simulink model "PIDkh4_controller"  (R2020a)
settings: Solver=VariableStepAuto  StartTime=0.0  StopTime=40  RelTol=1e-3
libraries: simulink x2, dspinverses x1
settings Model: Creator=FlightControlLab  LastModifiedBy=javier
settings SolverCC: SolverResetMethod=Robust
settings DataIOCC: ReturnWorkspaceOutputs=off
settings DebuggingCC: ArithmeticOperatorsInVariantConditions=warning
settings SFSimCC: SimUseLocalCustomCode=off  CustomCodeUndefinedFunction=UseInterfaceOnly
settings RTWCC: RTWUseLocalCustomCode=off

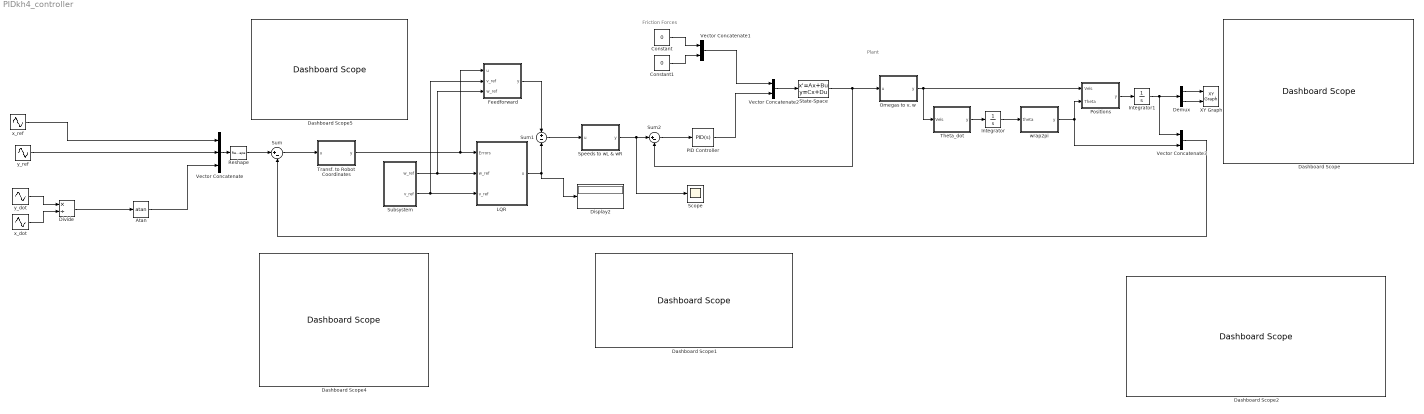
== system PIDkh4_controller ==
  note: Plant
  note: Friction Forces
  Atan : Trigonometry  Operator=atan
  Constant : Constant  Value=0
  Constant1 : Constant  Value=0
  Dashboard Scope{,1..2,4..5} (5 alike) : DashboardScope
  Demux : Demux  Outputs=2
  Display2 : Display
  Divide : Product  Inputs=*/
  Feedforward : MATLAB Function  TreatAsAtomicUnit=on
  Integrator : Integrator
  Integrator1 : Integrator
  LQR : Subsystem
  "Omegas to v, w" : MATLAB Function  TreatAsAtomicUnit=on
  PID Controller : simulink/Continuous/PID Controller  Controller=PID  Form=Parallel  TimeDomain=Continuous-time  UseExternalTs=off  SampleTime=-1  IntegratorMethod=Forward Euler  FilterMethod=Forward Euler  ControllerParametersSource=internal  P=10  I=10  D=1  UseFilter=on  N=100  TunerSelectOption=Transfer Function Based (PID Tuner App)  InitialConditionSource=internal  InitialConditionForIntegrator=0  InitialConditionForFilter=0  DifferentiatorICPrevScaledInput=0  ExternalReset=none  TrackingMode=off  Kt=1  LimitOutput=off  UpperSaturationLimit=inf  LowerSaturationLimit=-inf  LinearizeAsGain=on  AntiWindupMode=none  Kb=1  POutMin=[]  POutMax=[]  IOutMin=[]  IOutMax=[]  DOutMin=[]  DOutMax=[]  NOutMin=[]  NOutMax=[]  SumOutMin=[]  SumOutMax=[]  SaturationOutMin=[]  SaturationOutMax=[]  PParamMin=[]  PParamMax=[]  IParamMin=[]  IParamMax=[]  DParamMin=[]  DParamMax=[]  NParamMin=[]  NParamMax=[]  KbParamMin=[]  KbParamMax=[]  KtParamMin=[]  KtParamMax=[]  KbOutMin=[]  KbOutMax=[]  KtOutMin=[]  KtOutMax=[]  IntegratorOutMin=[]  IntegratorOutMax=[]  FilterOutMin=[]  FilterOutMax=[]  SumI1OutMin=[]  SumI1OutMax=[]  SumI2OutMin=[]  SumI2OutMax=[]  SumI3OutMin=[]  SumI3OutMax=[]  SumI4OutMin=[]  SumI4OutMax=[]  SumDOutMin=[]  SumDOutMax=[]  DifferentiatorOutMin=[]  DifferentiatorOutMax=[]  FilterDiffOutCoefMin=[]  FilterDiffOutCoefMax=[]  ReciprocalOutMin=[]  ReciprocalOutMax=[]  SumDenOutMin=[]  SumDenOutMax=[]  SumNumOutMin=[]  SumNumOutMax=[]  DivideOutMin=[]  DivideOutMax=[]  UdiffTsProdOutMin=[]  UdiffTsProdOutMax=[]  NTsProdOutMin=[]  NTsProdOutMax=[]  UintegralTsProdOutMin=[]  UintegralTsProdOutMax=[]  UngainTsProdOutMin=[]  UngainTsProdOutMax=[]  IntegratorContinuousStateAttributes=''  IntegratorStateMustResolveToSignalObject=off  IntegratorRTWStateStorageClass=Auto  FilterContinuousStateAttributes=''  FilterStateMustResolveToSignalObject=off  FilterRTWStateStorageClass=Auto  ParallelPVariant=InternalParameters  IdealPVariant=Disabled  IVariant=InternalParameters  DVariant=InternalParameters  IntegratorVariant=Continuous  SatVariant=Disabled  AWVariant=Passthrough  PCopyVariant=Disabled  TRVariant=Disabled  FdbkBlocksVariant=Forward  IdealPFdbkVariant=Disabled  SatFdbkVariant=Disabled  DerivativeFilterVariant=ContFilter  NVariant=InternalParameters  NCopyVariant=Disabled  FilterICVariant=InternalICsFilter  IntegratorICVariant=InternalICs  ExternalResetVariant=Disabled  TRSumVariant=Passthrough  SumFdbkVariant=Disabled  SumVariant=Sum_PID  TsampFilterVariant=InternalTs  TsampNgainVariant=Passthrough  TsampIntegralVariant=Passthrough
  Positions : MATLAB Function  TreatAsAtomicUnit=on
  Reshape : Reshape  OutputDimensionality=Column vector (2-D)
  Scope : Scope
  Speeds to wL & wR : MATLAB Function  TreatAsAtomicUnit=on
  State-Space : StateSpace  A=[0, 0, 0, 0; 0, 0, 0, 0; 0, 0, -0.0100, 0; 0, 0, 0, -0.0100]  B=[1.7699, 1.7699, 0, 0; 0.725, -0.725, 0, 0; -0.2100, 0, 10, 0; 0, -0.2100, 0, 10.0000]  C=[0, 0, 1, 0; 0, 0, 0, 1]  D=[0, 0, 0, 0; 0, 0, 0, 0]  InitialCondition=0
  Subsystem : Subsystem
  Sum : Sum  Inputs=|+-
  Sum1 : Sum  Inputs=+-
  Sum2 : Sum  Inputs=|+-
  Theta_dot : MATLAB Function  TreatAsAtomicUnit=on
  Transf. to Robot Coordinates : MATLAB Function  TreatAsAtomicUnit=on
  Vector Concatenate : Concatenate  NumInputs=3
  Vector Concatenate1 : Concatenate
  Vector Concatenate2 : Concatenate
  Vector Concatenate3 : Concatenate
  XY Graph : simulink/Sinks/XY Graph  xmin=-1  xmax=1  ymin=-1  ymax=1  st=-1
  wrap2pi : MATLAB Function  TreatAsAtomicUnit=on
  x_dot : Sin  Amplitude=0.3^2  Frequency=0.3  Phase=pi/2  SampleTime=0
  x_ref : Sin  Amplitude=0.3  Frequency=0.3  SampleTime=0
  y_dot : Sin  Amplitude=-0.3^2  Frequency=0.3  SampleTime=0
  y_ref : Sin  Amplitude=0.3  Bias=-0.3  Frequency=0.3  Phase=pi/2  SampleTime=0
  wires:
  x_ref/1 -> Vector Concatenate/1
  y_ref/1 -> Vector Concatenate/2
  Transf. to Robot Coordinates/1(y) -> LQR/1(Errors), Feedforward/1(u)
  Subsystem/1(w_ref) -> LQR/2(w_ref), Feedforward/3(w_ref)
  Sum1/1 -> Speeds to wL & wR/1(u)
  State-Space/1 -> Sum2/2, "Omegas to v, w"/1(u)
  Constant/1 -> Vector Concatenate1/1
  Constant1/1 -> Vector Concatenate1/2
  Vector Concatenate2/1 -> State-Space/1
  Vector Concatenate1/1 -> Vector Concatenate2/1
  Positions/1(y) -> Integrator1/1
  "Omegas to v, w"/1(y) -> Positions/1(Vels), Theta_dot/1(Vels)
  Theta_dot/1(y) -> Integrator/1
  Integrator1/1 -> Vector Concatenate3/1, Demux/1
  Vector Concatenate3/1 -> Sum/2
  Subsystem/2(v_ref) -> LQR/3(v_ref), Feedforward/2(v_ref)
  Vector Concatenate/1 -> Reshape/1
  Reshape/1 -> Sum/1
  Sum/1 -> Transf. to Robot Coordinates/1(u)
  Feedforward/1(y) -> Sum1/1
  y_dot/1 -> Divide/1
  x_dot/1 -> Divide/2
  Speeds to wL & wR/1(y) -> Scope/1, Sum2/1
  Sum2/1 -> PID Controller/1
  PID Controller/1 -> Vector Concatenate2/2
  LQR/1(u) -> Display2/1, Sum1/2
  Demux/1 -> XY Graph/1
  Demux/2 -> XY Graph/2
  Integrator/1 -> wrap2pi/1(theta)
  wrap2pi/1(y) -> Positions/2(Theta), Vector Concatenate3/2
  Atan/1 -> Vector Concatenate/3
  Divide/1 -> Atan/1

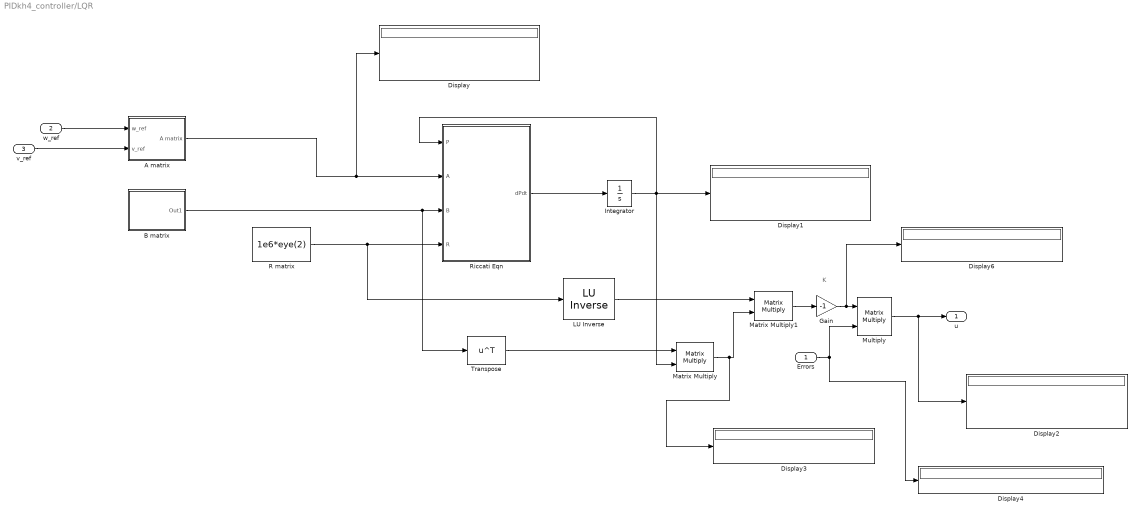
== system PIDkh4_controller/LQR ==
  note: K
  Errors : Inport
  w_ref : Inport  Port=2
  v_ref : Inport  Port=3
  " LU Inverse" : dspinverses/ LU Inverse
  A matrix : Subsystem
  B matrix : Subsystem
  Display{,1..4,6} (6 alike) : Display
  Gain : Gain  Gain=-1
  Integrator : Integrator
  Matrix Multiply : Product  Multiplication=Matrix(*)
  Matrix Multiply1 : Product  Multiplication=Matrix(*)
  Multiply : Product  Multiplication=Matrix(*)
  R matrix : Constant  Value=1e6*eye(2)  VectorParams1D=off
  Riccati Eqn : MATLAB Function  TreatAsAtomicUnit=on
  Transpose : Math  Operator=transpose  SignedPower=on  SaturateOnIntegerOverflow=on
  u : Outport  VectorParamsAs1DForOutWhenUnconnected=off
  wires:
  B matrix/1(Out1) -> Transpose/1, Riccati Eqn/3(B)
  R matrix/1 -> " LU Inverse"/1, Riccati Eqn/4(R)
  A matrix/1(A matrix) -> Display/1, Riccati Eqn/2(A)
  Multiply/1 -> Display2/1, u/1
  Integrator/1 -> Riccati Eqn/1(P), Display1/1, Matrix Multiply/2
  Matrix Multiply/1 -> Display3/1, Matrix Multiply1/2
  Transpose/1 -> Matrix Multiply/1
  Riccati Eqn/1(dPdt) -> Integrator/1
  w_ref/1 -> A matrix/1(w_ref)
  v_ref/1 -> A matrix/2(v_ref)
  Errors/1 -> Multiply/2, Display4/1
  " LU Inverse"/1 -> Matrix Multiply1/1
  Matrix Multiply1/1 -> Gain/1
  Gain/1 -> Display6/1, Multiply/1

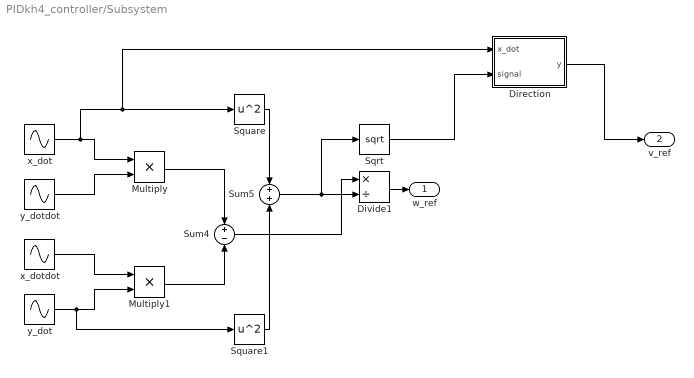
== system PIDkh4_controller/Subsystem ==
  Direction : MATLAB Function  TreatAsAtomicUnit=on
  Divide1 : Product  Inputs=*/
  Multiply : Product
  Multiply1 : Product
  Sqrt : Sqrt  SaturateOnIntegerOverflow=on
  Square : Math  Operator=square  SignedPower=on  SaturateOnIntegerOverflow=on
  Square1 : Math  Operator=square  SignedPower=on  SaturateOnIntegerOverflow=on
  Sum4 : Sum  Inputs=+-
  Sum5 : Sum
  x_dot : Sin  Amplitude=0.3^2  Frequency=0.3  Phase=pi/2  SampleTime=0
  x_dotdot : Sin  Amplitude=-0.3^3  Frequency=0.3  SampleTime=0
  y_dot : Sin  Amplitude=-0.3^2  Frequency=0.3  SampleTime=0
  y_dotdot : Sin  Amplitude=-0.3^3  Frequency=0.3  Phase=pi/2  SampleTime=0
  w_ref : Outport  VectorParamsAs1DForOutWhenUnconnected=off
  v_ref : Outport  Port=2  VectorParamsAs1DForOutWhenUnconnected=off
  wires:
  x_dot/1 -> Direction/1(x_dot), Square/1, Multiply/1
  Divide1/1 -> w_ref/1
  x_dotdot/1 -> Multiply1/1
  Sum5/1 -> Divide1/2, Sqrt/1
  Square/1 -> Sum5/1
  Sum4/1 -> Divide1/1
  y_dot/1 -> Square1/1, Multiply1/2
  y_dotdot/1 -> Multiply/2
  Multiply1/1 -> Sum4/2
  Square1/1 -> Sum5/2
  Multiply/1 -> Sum4/1
  Sqrt/1 -> Direction/2(signal)
  Direction/1(y) -> v_ref/1

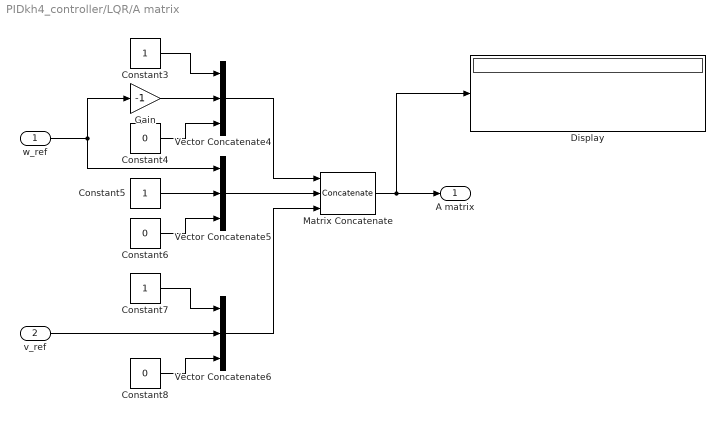
== system PIDkh4_controller/LQR/A matrix ==
  w_ref : Inport
  v_ref : Inport  Port=2
  Constant3 : Constant
  Constant4 : Constant  Value=0
  Constant5 : Constant
  Constant6 : Constant  Value=0
  Constant7 : Constant
  Constant8 : Constant  Value=0
  Display : Display
  Gain : Gain  Gain=-1
  Matrix Concatenate : Concatenate  NumInputs=3  Mode=Multidimensional array  ConcatenateDimension=2
  Vector Concatenate4 : Concatenate  NumInputs=3
  Vector Concatenate5 : Concatenate  NumInputs=3
  Vector Concatenate6 : Concatenate  NumInputs=3
  A matrix : Outport  VectorParamsAs1DForOutWhenUnconnected=off
  wires:
  w_ref/1 -> Gain/1, Vector Concatenate5/1
  Gain/1 -> Vector Concatenate4/2
  Constant6/1 -> Vector Concatenate5/3
  Vector Concatenate6/1 -> Matrix Concatenate/3
  Constant4/1 -> Vector Concatenate4/3
  v_ref/1 -> Vector Concatenate6/2
  Constant7/1 -> Vector Concatenate6/1
  Vector Concatenate5/1 -> Matrix Concatenate/2
  Constant8/1 -> Vector Concatenate6/3
  Constant3/1 -> Vector Concatenate4/1
  Constant5/1 -> Vector Concatenate5/2
  Vector Concatenate4/1 -> Matrix Concatenate/1
  Matrix Concatenate/1 -> Display/1, A matrix/1

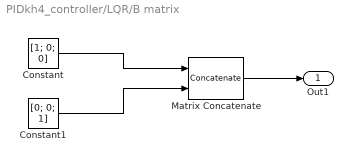
== system PIDkh4_controller/LQR/B matrix ==
  Constant : Constant  Value=[1; 0; 0]  VectorParams1D=off
  Constant1 : Constant  Value=[0; 0; 1]  VectorParams1D=off
  Matrix Concatenate : Concatenate  Mode=Multidimensional array  ConcatenateDimension=2
  Out1 : Outport  VectorParamsAs1DForOutWhenUnconnected=off
  wires:
  Constant/1 -> Matrix Concatenate/1
  Matrix Concatenate/1 -> Out1/1
  Constant1/1 -> Matrix Concatenate/2

== matlab function PIDkh4_controller/Subsystem/Direction ==
  data: x_dot input; y output; signal input
function y = fcn(x_dot, signal)
if x_dot < 0
    y = -signal;
else
    y = signal;
end
end

== matlab function PIDkh4_controller/Transf. to Robot Coordinates ==
  data: u input size=[3,1]; y output size=[3,1]
function y = fcn(u)

theta = u(3);
A = [cos(theta), sin(theta), 0;
    -sin(theta), cos(theta), 0;
    0, 0, 1];

y = A*u;

== matlab function PIDkh4_controller/Feedforward ==
  data: u input size=[3,1]; y output size=[2,1]; v_ref input size=1; w_ref input size=1
function y = fcn(u, v_ref, w_ref)

    e3 = u(3);
    
    y = [cos(e3)*v_ref;
        w_ref];

== matlab function PIDkh4_controller/Speeds to wL & wR ==
  data: u input size=2; y output size=2
function y = fcn(u)

r = 0.021; % Wheel radius
D = 0.145; % Robot diameter

v = u(1);
w = u(2);

v_r = (2*v+w*D)/2;
v_l = (2*v-w*D)/2;

w_l = v_l/r;
w_r = v_r/r;

y =  [w_l;
    w_r];

== matlab function PIDkh4_controller/Theta_dot ==
  data: Vels input size=2; y output size=1
function y = fcn(Vels)

y = Vels(2);

== matlab function PIDkh4_controller/Positions ==
  data: Vels input size=2; Theta input size=1; y output size=2
function y = fcn(Vels, Theta)

v = Vels(1);

x1 = v * cos(Theta);
x2 = v * sin(Theta);

y = [x1; x2];

== matlab function PIDkh4_controller/Omegas to v, w ==
  data: u input size=2; y output size=2
function y = fcn(u)
r = 0.021; % Wheel radius
D = 0.145; % Robot diameter

v = u*r; 

v_l = v(1);
v_r = v(2);

omega = (v_r - v_l)/D;
v = (v_r + v_l)/2;

y = [v; omega];

== matlab function PIDkh4_controller/LQR/Riccati Eqn ==
  data: dPdt output size=[3,3]; P input size=[3,3]; A input size=[3,3]; B input size=[3,2]; R input size=[2,2]
function dPdt = mRiccati(P,A,B,R)

% A = rand(3,3);
% B = rand(3,2);
Q = diag([1 1 10]);
% R = 1e-4*diag([1 1]);
% P = rand(3,3);


% Continuous Riccati differential equation
dPdt = -(A'*P + P*A - (P*B)*pinv(R)*(B'*P) + Q);

== matlab function PIDkh4_controller/wrap2pi ==
  data: theta input; y output
function y = fcn(theta)
y = theta;
if theta <= -pi/2
    y = theta + pi;
elseif theta > pi/2
    y = theta - pi;
end
